simulink model "HallSensor"  (R2023a)
settings: Solver=VariableStepAuto  StartTime=0.0  StopTime=10.0  RelTol=1e-3
settings Model: Creator=Сафроновы  LastModifiedBy=Сафроновы

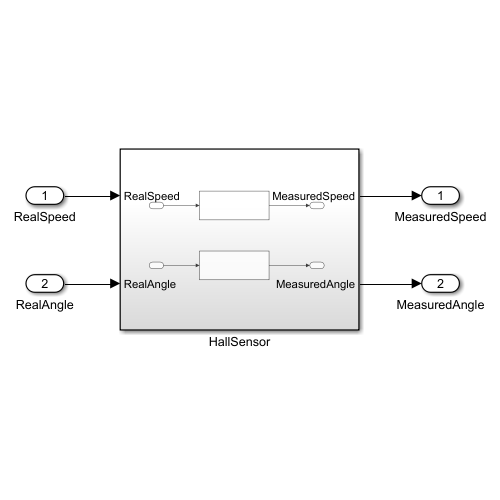
[thumbnail: Simulink's stored preview of the top-level diagram]
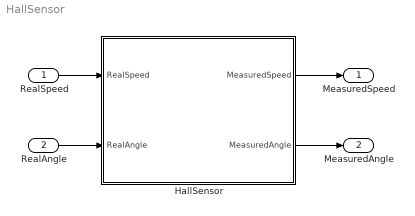
== system HallSensor ==
  RealSpeed : Inport
  RealAngle : Inport  Port=2
  HallSensor : Subsystem
  MeasuredSpeed : Outport
  MeasuredAngle : Outport  Port=2
  wires:
  RealSpeed/1 -> HallSensor/1(RealSpeed)
  RealAngle/1 -> HallSensor/2(RealAngle)
  HallSensor/1(MeasuredSpeed) -> MeasuredSpeed/1
  HallSensor/2(MeasuredAngle) -> MeasuredAngle/1

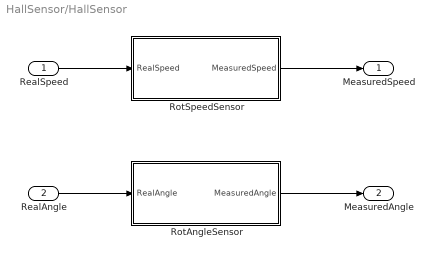
== system HallSensor/HallSensor ==
  RealSpeed : Inport
  RealAngle : Inport  Port=2
  RotAngleSensor : Subsystem
  RotSpeedSensor : Subsystem
  MeasuredSpeed : Outport
  MeasuredAngle : Outport  Port=2
  wires:
  RotSpeedSensor/1(MeasuredSpeed) -> MeasuredSpeed/1
  RealAngle/1 -> RotAngleSensor/1(RealAngle)
  RealSpeed/1 -> RotSpeedSensor/1(RealSpeed)
  RotAngleSensor/1(MeasuredAngle) -> MeasuredAngle/1

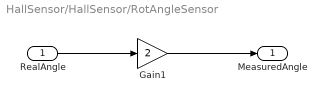
== system HallSensor/HallSensor/RotAngleSensor ==
  RealAngle : Inport
  Gain1 : Gain  Gain=2
  MeasuredAngle : Outport
  wires:
  Gain1/1 -> MeasuredAngle/1
  RealAngle/1 -> Gain1/1

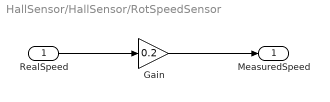
== system HallSensor/HallSensor/RotSpeedSensor ==
  RealSpeed : Inport
  Gain : Gain  Gain=0.2
  MeasuredSpeed : Outport
  wires:
  RealSpeed/1 -> Gain/1
  Gain/1 -> MeasuredSpeed/1
